simulink model "dynamicModel"  (R2019b)
settings: Solver=VariableStepAuto  StartTime=0.0  StopTime=8  RelTol=1e-6
values from neighbouring files (symbols this model uses):
  P = 4    [dq_3hp_induction.m]
  rs = 0.45    [dq_3hp_induction.m]
  wb = 2*pi*f    (= 376.991118431)    [dq_3hp_induction.m]
undefined symbols (not defined in the file or in its folder): rr_prime, V, Xlr_prime, Xls, Xm
libraries: simulink x5
settings Model: Creator=t_sta  LastModifiedBy=carlo
settings DataIOCC: ReturnWorkspaceOutputs=off
settings DebuggingCC: ArithmeticOperatorsInVariantConditions=warning
settings SFSimCC: SimUseLocalCustomCode=off  CustomCodeUndefinedFunction=UseInterfaceOnly
settings RTWCC: RTWUseLocalCustomCode=off

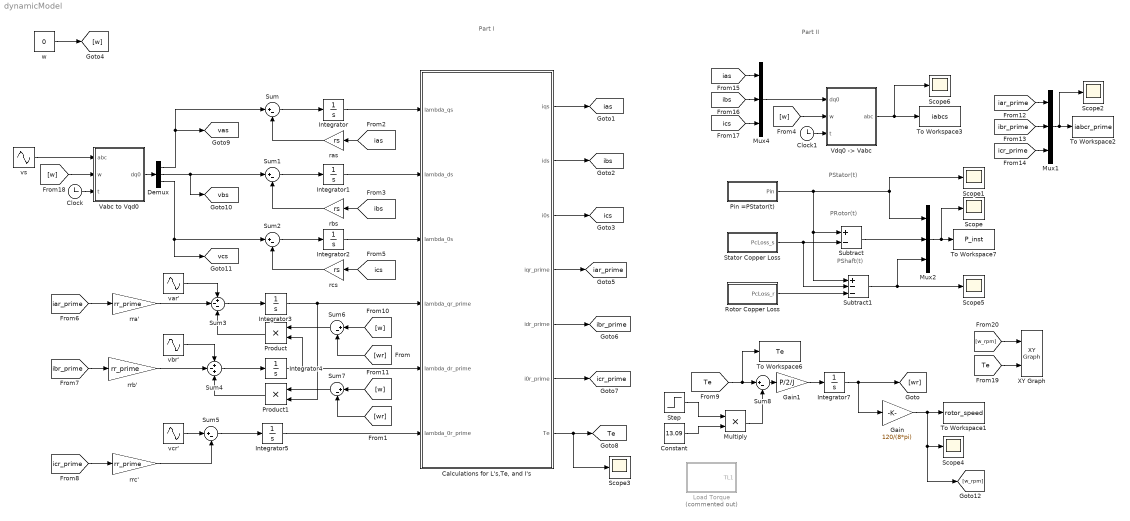
== system dynamicModel ==
  note: PShaft(t)
  note: Part I
  note: Part II
  note: PRotor(t)
  note: PStator(t)
  "Calculations for L's,Te, and I's" : MATLAB Function  TreatAsAtomicUnit=on
  Clock : Clock
  Clock1 : Clock
  Constant : Constant  Value=13.09
  Demux : Demux  Outputs=3
  Gain : Gain  Gain=120/(8*pi)
  Gain1 : Gain  Gain=P/2/J
  Integrator{,1..5,7} (7 alike) : Integrator
  Load Torque : Subsystem  Commented=on
  Multiply : Product
  Mux1 : Mux  Inputs=3
  Mux2 : Mux  Inputs=3
  Mux4 : Mux  Inputs=3
  Pin =PStator(t) : Subsystem
  Product : Product
  Product1 : Product
  Rotor Copper Loss : Subsystem
  Scope{,1..6} (7 alike) : Scope
  Stator Copper Loss : Subsystem
  Step : Step  Time=0.5  SampleTime=0
  Subtract : Sum  Inputs=+-
  Subtract1 : Sum  Inputs=+--
  Sum{,1..2,5..8} (7 alike) : Sum  Inputs=|+-
  Sum3 : Sum  Inputs=+--
  Sum4 : Sum  Inputs=+-+
  To Workspace1 : ToWorkspace  VariableName=rotor_speed  SaveFormat=Structure With Time  SampleTime=-1
  To Workspace2 : ToWorkspace  VariableName=iabcr_prime  SaveFormat=Structure With Time  SampleTime=-1
  To Workspace3 : ToWorkspace  VariableName=iabcs  SaveFormat=Structure With Time  SampleTime=-1
  To Workspace6 : ToWorkspace  VariableName=Te  SaveFormat=Structure With Time  SampleTime=-1
  To Workspace7 : ToWorkspace  VariableName=P_inst  SaveFormat=Structure With Time  SampleTime=-1
  Vabc to Vqd0 : MATLAB Function  TreatAsAtomicUnit=on
  "Vdq0 -> Vabc" : MATLAB Function  TreatAsAtomicUnit=on
  XY Graph : simulink/Sinks/XY Graph  xmin=0  xmax=3900  ymin=-60  ymax=180  st=-1
  ras : Gain  Gain=rs
  rbs : Gain  Gain=rs
  rcs : Gain  Gain=rs
  rra' : Gain  Gain=rr_prime
  rrb' : Gain  Gain=rr_prime
  rrc' : Gain  Gain=rr_prime
  var' : Sin  Amplitude=0  Frequency=377  SampleTime=0
  vbr' : Sin  Amplitude=0  Frequency=377  Phase=-2*pi/3  SampleTime=0
  vcr' : Sin  Amplitude=0  Frequency=377  Phase=2*pi/3  SampleTime=0
  vs : Sin  Amplitude=V  Frequency=wb  Phase=[0 -1 1]*2*pi/3  SampleTime=0
  w : Constant  Value=0
  tag scope: Te=global, iar_prime=global, ias=global, ibr_prime=global, ibs=global, icr_prime=global, ics=global, vas=global, vbs=global, vcs=global
  wires:
  rrc'/1 -> Sum5/2
  rcs/1 -> Sum2/2
  rrb'/1 -> Sum4/2
  Sum4/1 -> Integrator4/1
  vbr'/1 -> Sum4/1
  Sum2/1 -> Integrator2/1
  Sum5/1 -> Integrator5/1
  Sum1/1 -> Integrator1/1
  ras/1 -> Sum/2
  var'/1 -> Sum3/1
  Sum/1 -> Integrator/1
  vcr'/1 -> Sum5/1
  rra'/1 -> Sum3/2
  rbs/1 -> Sum1/2
  Sum3/1 -> Integrator3/1
  "Calculations for L's,Te, and I's"/1(iqs) -> [ias]
  "Calculations for L's,Te, and I's"/2(ids) -> [ibs]
  "Calculations for L's,Te, and I's"/3(i0s) -> [ics]
  "Calculations for L's,Te, and I's"/4(iqr_prime) -> [iar_prime]
  "Calculations for L's,Te, and I's"/5(idr_prime) -> [ibr_prime]
  "Calculations for L's,Te, and I's"/6(i0r_prime) -> [icr_prime]
  [ias] -> ras/1
  [ibs] -> rbs/1
  [ics] -> rcs/1
  [iar_prime] -> rra'/1
  [ibr_prime] -> rrb'/1
  [icr_prime] -> rrc'/1
  "Calculations for L's,Te, and I's"/7(Te) -> [Te], Scope3/1
  Gain/1 -> [w_rpm], Scope4/1, To Workspace1/1
  Gain1/1 -> Integrator7/1
  Integrator7/1 -> [wr], Gain/1
  Mux1/1 -> Scope2/1, To Workspace2/1
  Mux2/1 -> To Workspace7/1, Scope/1
  Subtract/1 -> Mux2/2
  Pin =PStator(t)/1(Pin) -> Scope1/1, Mux2/1, Subtract1/1, Subtract/1
  Stator Copper Loss/1(PcLoss_s) -> Subtract1/2, Subtract/2
  Rotor Copper Loss/1(PcLoss_r) -> Subtract1/3
  Subtract1/1 -> Scope5/1, Mux2/3
  Vabc to Vqd0/1(dq0) -> Demux/1
  Demux/1 -> Sum/1, [vas]
  Demux/2 -> [vbs], Sum1/1
  Demux/3 -> Sum2/1, [vcs]
  [w] -> Vabc to Vqd0/2(w)
  Clock/1 -> Vabc to Vqd0/3(t)
  Integrator/1 -> "Calculations for L's,Te, and I's"/1(lambda_qs)
  Integrator1/1 -> "Calculations for L's,Te, and I's"/2(lambda_ds)
  Integrator2/1 -> "Calculations for L's,Te, and I's"/3(lambda_0s)
  Integrator3/1 -> Product1/2, "Calculations for L's,Te, and I's"/4(lambda_qr_prime)
  Integrator4/1 -> "Calculations for L's,Te, and I's"/5(lambda_dr_prime), Product/2
  Integrator5/1 -> "Calculations for L's,Te, and I's"/6(lambda_0r_prime)
  "Vdq0 -> Vabc"/1(abc) -> Scope6/1, To Workspace3/1
  [w] -> "Vdq0 -> Vabc"/2(w)
  Clock1/1 -> "Vdq0 -> Vabc"/3(t)
  Product/1 -> Sum3/3
  Sum6/1 -> Product/1
  [wr] -> Sum6/2
  [w] -> Sum6/1
  [w] -> Sum7/1
  [wr] -> Sum7/2
  Product1/1 -> Sum4/3
  [Te] -> Sum8/1, To Workspace6/1
  Sum8/1 -> Gain1/1
  Multiply/1 -> Sum8/2
  w/1 -> [w]
  Sum7/1 -> Product1/1
  [iar_prime] -> Mux1/1
  [ibr_prime] -> Mux1/2
  [icr_prime] -> Mux1/3
  [ics] -> Mux4/3
  [ibs] -> Mux4/2
  [ias] -> Mux4/1
  Mux4/1 -> "Vdq0 -> Vabc"/1(dq0)
  vs/1 -> Vabc to Vqd0/1(abc)
  Step/1 -> Multiply/1
  Constant/1 -> Multiply/2
  [Te] -> XY Graph/2
  [w_rpm] -> XY Graph/1

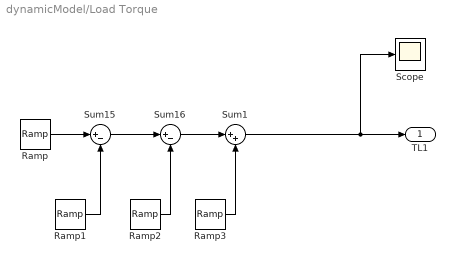
== system dynamicModel/Load Torque ==
  Ramp : simulink/Sources/Ramp  slope=0.25*52.36/2  start=2  InitialOutput=0
  Ramp1 : simulink/Sources/Ramp  slope=0.25*52.36/2  start=4  InitialOutput=0
  Ramp2 : simulink/Sources/Ramp  slope=0.25*52.36/2  start=6  InitialOutput=0
  Ramp3 : simulink/Sources/Ramp  slope=0.25*52.36/2  start=8  InitialOutput=0
  Scope : Scope
  Sum1 : Sum  Inputs=|++
  Sum15 : Sum  Inputs=|+-
  Sum16 : Sum  Inputs=|+-
  TL1 : Outport  VectorParamsAs1DForOutWhenUnconnected=off
  wires:
  Ramp/1 -> Sum15/1
  Ramp1/1 -> Sum15/2
  Sum15/1 -> Sum16/1
  Ramp2/1 -> Sum16/2
  Sum16/1 -> Sum1/1
  Sum1/1 -> Scope/1, TL1/1
  Ramp3/1 -> Sum1/2

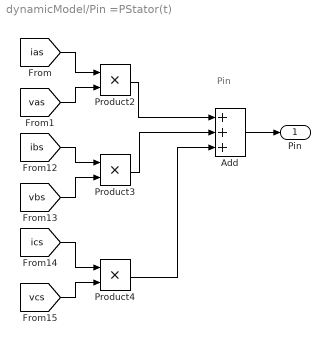
== system dynamicModel/Pin =PStator(t) ==
  note: Pin
  Add : Sum  Inputs=+++
  Product2 : Product  RndMeth=Zero
  Product3 : Product  RndMeth=Zero
  Product4 : Product  RndMeth=Zero
  Pin : Outport  VectorParamsAs1DForOutWhenUnconnected=off
  wires:
  [ics] -> Product4/1
  [vas] -> Product2/2
  Product3/1 -> Add/2
  Product4/1 -> Add/3
  [vbs] -> Product3/2
  [ibs] -> Product3/1
  Product2/1 -> Add/1
  [ias] -> Product2/1
  [vcs] -> Product4/2
  Add/1 -> Pin/1

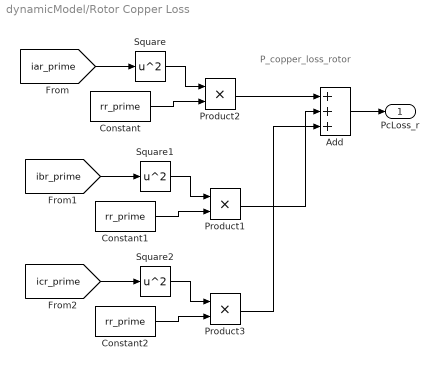
== system dynamicModel/Rotor Copper Loss ==
  note: P_copper_loss_rotor
  Add : Sum  Inputs=+++
  Constant : Constant  Value=rr_prime
  Constant1 : Constant  Value=rr_prime
  Constant2 : Constant  Value=rr_prime
  Product1 : Product  RndMeth=Zero
  Product2 : Product  RndMeth=Zero
  Product3 : Product  RndMeth=Zero
  Square : Math  Operator=square  SaturateOnIntegerOverflow=on
  Square1 : Math  Operator=square  SaturateOnIntegerOverflow=on
  Square2 : Math  Operator=square  SaturateOnIntegerOverflow=on
  PcLoss_r : Outport  VectorParamsAs1DForOutWhenUnconnected=off
  wires:
  Product2/1 -> Add/1
  Add/1 -> PcLoss_r/1
  Constant/1 -> Product2/2
  [iar_prime] -> Square/1
  Square/1 -> Product2/1
  [ibr_prime] -> Square1/1
  Square1/1 -> Product1/1
  Constant1/1 -> Product1/2
  Product1/1 -> Add/2
  [icr_prime] -> Square2/1
  Square2/1 -> Product3/1
  Constant2/1 -> Product3/2
  Product3/1 -> Add/3

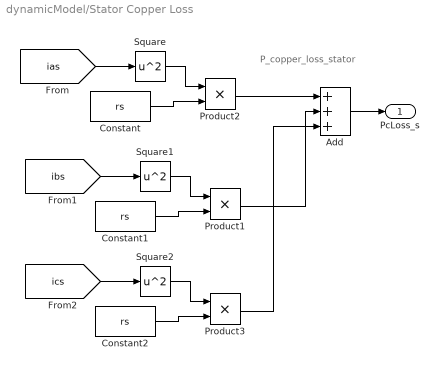
== system dynamicModel/Stator Copper Loss ==
  note: P_copper_loss_stator
  Add : Sum  Inputs=+++
  Constant : Constant  Value=rs
  Constant1 : Constant  Value=rs
  Constant2 : Constant  Value=rs
  Product1 : Product  RndMeth=Zero
  Product2 : Product  RndMeth=Zero
  Product3 : Product  RndMeth=Zero
  Square : Math  Operator=square  SaturateOnIntegerOverflow=on
  Square1 : Math  Operator=square  SaturateOnIntegerOverflow=on
  Square2 : Math  Operator=square  SaturateOnIntegerOverflow=on
  PcLoss_s : Outport  VectorParamsAs1DForOutWhenUnconnected=off
  wires:
  Product2/1 -> Add/1
  Add/1 -> PcLoss_s/1
  Constant/1 -> Product2/2
  [ias] -> Square/1
  Square/1 -> Product2/1
  [ibs] -> Square1/1
  Square1/1 -> Product1/1
  Constant1/1 -> Product1/2
  Product1/1 -> Add/2
  [ics] -> Square2/1
  Square2/1 -> Product3/1
  Constant2/1 -> Product3/2
  Product3/1 -> Add/3

== matlab function dynamicModel/Calculations for L's,Te, and I's ==
  data: lambda_qs input; lambda_ds input; iqs output; lambda_0s input; lambda_qr_prime input; lambda_dr_prime input; lambda_0r_prime input; ids output; i0s output; iqr_prime output; idr_prime output; i0r_prime output; Te output; P parameter; Xls parameter; Xlr_prime parameter; Xm parameter; wb parameter
function [iqs, ids, i0s, iqr_prime, idr_prime, i0r_prime, Te] = fcn(lambda_qs, lambda_ds, lambda_0s, lambda_qr_prime, lambda_dr_prime, lambda_0r_prime, P, Xls, Xlr_prime, Xm, wb)

LM = Xm/wb;
Lls = Xls/wb;
Llr_prime = Xlr_prime/wb;

Ks_Ls_Ksinv = [ Lls+LM, 0, 0;
                0, Lls+LM, 0;
                0, 0, Lls+LM];

Kr_L_prime_r_Krinv = [Llr_prime+LM, 0, 0; 0, Llr_prime+LM, 0; 0, 0, Llr_prime];

Kr_L_prime_sr_Ksinv = [LM, 0, 0; 0, LM, 0; 0, 0, 0];

L = [Ks_Ls_Ksinv, Kr_L_prime_sr_Ksinv; Kr_L_prime_sr_Ksinv, Kr_L_prime_r_Krinv];

lambda = [lambda_qs; lambda_ds; lambda_0s; lambda_qr_prime; lambda_dr_prime; lambda_0r_prime];

I = L\lambda;

%Extract Individual Currents
iqs = I(1);
ids = I(2);
i0s = I(3);
iqr_prime = I(4);
idr_prime = I(5);
i0r_prime = I(6);

%Calculate Load Torque
Te = (3/2)*(P/2)*(lambda_ds*iqs - lambda_qs*ids);

== matlab function dynamicModel/Vabc to Vqd0 ==
  data: abc input; w input; dq0 output; t input
function dq0 = fcn(abc, w, t)
    ks = ((2/3)*[cos(w*t) cos(w*t - (2*pi/3)) cos(w*t + (2*pi/3)); 
        sin(w*t) sin(w*t - (2*pi/3)) sin(w*t + (2*pi/3)); 
        (1/2) (1/2) (1/2)]);
   dq0 = ks*abc; 
   
end

== matlab function dynamicModel/Vdq0 -> Vabc ==
  data: dq0 input; w input; abc output; t input
function abc = fcn(dq0, w, t)
    ks_inverse = [cos(w*t) sin(w*t) 1;
        cos(w*t - (2*pi/3)) sin(w*t - (2*pi/3)) 1;
        cos(w*t + (2*pi/3)) sin(w*t + (2*pi/3)) 1];
    
   abc = ks_inverse*dq0; 
   
end
